simulink model "diastaurosh_31_10_servo_angle"  (R2024b)
settings: Solver=FixedStepDiscrete  StartTime=0.0  StopTime=inf  FixedStep=0.00001  RelTol=1e-3  EnableMultiTasking=on
undefined symbols (not defined in the file): DiscIntNeverNeededParam
libraries: frdmtfcshieldlib x8, slpidlib x4, RHIT_KL25Z_Library x2, Autonomous_Vehicle_Competition x2, frdmkl25zlib x2
settings Model: Creator=maste  LastModifiedBy=kapki
settings SolverCC: AutoInsertRateTranBlk=on  EnableFixedStepZeroCrossing=on
settings DataIOCC: ReturnWorkspaceOutputs=off
settings OptimizationCC: LifeSpan=1  MaxStackSize=64  EfficientTunableParamExpr=on
settings DebuggingCC: ArithmeticOperatorsInVariantConditions=warning
settings HardwareCC: ProdBitPerPointer=32  ProdBitPerSizeT=32  ProdBitPerPtrDiffT=32  ProdLargestAtomicInteger=Long  ProdLargestAtomicFloat=Double  ProdWordSize=32  ProdHWDeviceType=ARM Compatible->ARM Cortex
settings ModelReferenceCC: EnableRefExpFcnMdlSchedulingChecks=on
settings SFSimCC: MATLABDynamicMemAlloc=off  CustomCodeUndefinedFunction=UseInterfaceOnly
settings RTWCC: Description=Embedded Coder  SystemTargetFile=ert.tlc  HardwareBoard=NXP FRDM-KL25Z  TemplateMakefile=ert_default_tmf  Toolchain=GNU Tools for ARM Embedded Processors  GPUComputeCapability=3.5
settings CodeAppCC: IgnoreCustomStorageClasses=off  StateflowObjectComments=on
settings ERTTargetCC: MultiwordLength=2048  SupportContinuousTime=on  InlinedParameterPlacement=Hierarchical  ConvertIfToSwitch=off  SuppressUnreachableDefaultCases=off  DynamicArrayContainerType=coder::array

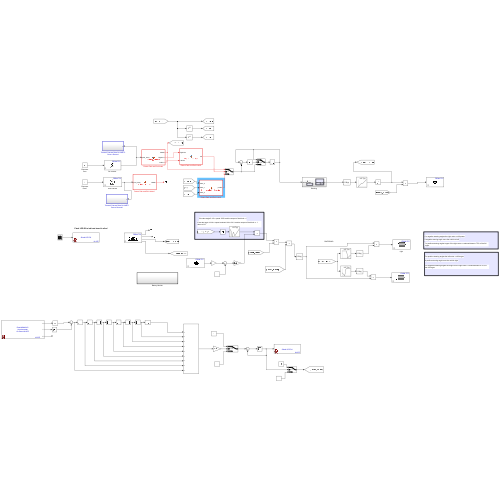
[thumbnail: Simulink's stored preview of the top-level diagram]
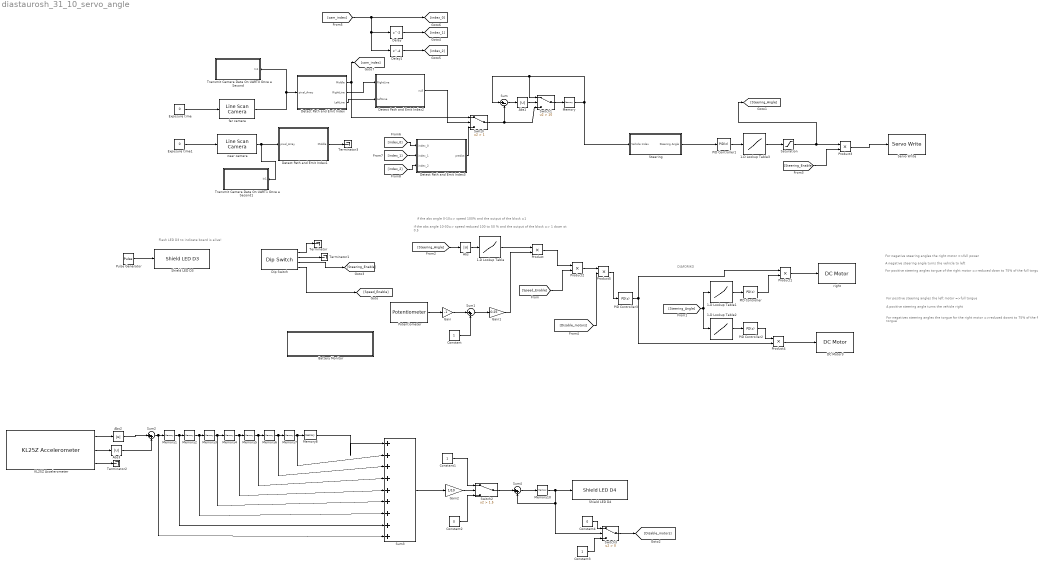
== system diastaurosh_31_10_servo_angle ==
  note: Flash LED D3 to indicate board is alive!
  note: if the abs angle 0-10=> speed 100% and the output of the block =1
  note: if the abs angle 10-30=> speed reduced 100 to 50 % and the output of the block => 1 down ot 0.5
  note: For positive steering angles torgue of the right motor =>reduced down to 75% of the full torgue
  note: For negatives steering angles the torgue for the right motor =>reduced downt to 75% of the full torgue
  note: For positive steering angles the left motor =>full torgue
  note: For negative steering angles the right motor =>full power
  note: A negative steering angle turns the vehicle to left
  note: DIAFORIKO
  note: A positive steering angle turns the vehicle right
  1-D Lookup Table : Lookup_n-D  NumberOfTableDimensions=1  BreakpointsForDimension1="[0  10 20 30 60]"  Table=[ 1.4 0.9 1.2 0.95 1.4]  ExtrapMethod=Clip  UseLastTableValue=on  InternalRulePriority=Speed  RndMeth=Simplest
  1-D Lookup Table1 : Lookup_n-D  NumberOfTableDimensions=1  BreakpointsForDimension1=[-60 0 10 20 60]  Table=[1.1 1.1 1 0.6 0.8]  ExtrapMethod=Clip  UseLastTableValue=on  InternalRulePriority=Speed  RndMeth=Simplest
  1-D Lookup Table2 : Lookup_n-D  NumberOfTableDimensions=1  BreakpointsForDimension1="[-60  -20 -10  0 60]"  Table=[0.8 0.6 1 1.1 1.1]  ExtrapMethod=Clip  UseLastTableValue=on  InternalRulePriority=Speed  RndMeth=Simplest
  1-D Lookup Table3 : Lookup_n-D  NumberOfTableDimensions=1  BreakpointsForDimension1=[-60 -9 9 60]  Table=[-60 0 0 60]  ExtrapMethod=Clip  UseLastTableValue=on  InternalRulePriority=Speed  RndMeth=Simplest
  Abs{,1..3} (4 alike) : Abs  SaturateOnIntegerOverflow=off
  Battery Monitor : Subsystem  TreatAsAtomicUnit=on  SystemSampleTime=0.1
  Constant : Constant
  Constant1 : Constant
  Constant2 : Constant  Value=0
  Constant3 : Constant
  Constant4 : Constant  Value=0
  DC Motor3 : frdmtfcshieldlib/DC Motor  WhichMotor=B
  Delay : Delay  InitialCondition=64
  Delay1 : Delay  DelayLength=4  InitialCondition=64
  Detect Path and Emit Index : MATLAB Function  TreatAsAtomicUnit=on
  Detect Path and Emit Index1 : MATLAB Function  TreatAsAtomicUnit=on
  Detect Path and Emit Index2 : MATLAB Function  TreatAsAtomicUnit=on
  Detect Path and Emit Index3 : MATLAB Function  TreatAsAtomicUnit=on
  Dip Switch : frdmtfcshieldlib/Dip Switch  SampleTime=-1
  Exposure time : Constant  Value=0
  Exposure time1 : Constant  Value=0
  Gain : Gain  Gain=-1
  Gain1 : Gain  Gain=0.25
  Gain2 : Gain  Gain=1/10
  KL25Z Accelerometer : RHIT_KL25Z_Library/Sensor Read Functions/KL25Z Accelerometer
      settings: SourceProductName=RHIT KL25Z Library
  Memory : Memory  InitialCondition=64
  Memory{1..8,10} (9 alike) : Memory
  PID Controller : slpidlib/PID Controller  Controller=PD  Form=Parallel  TimeDomain=Discrete-time  UseExternalTs=off  SampleTime=-1  IntegratorMethod=Forward Euler  FilterMethod=Forward Euler  ControllerParametersSource=internal  P=1  I=1  UseKiTs=off  D=0  UseExternalDerivativeSource=off  N=100  UseFilter=on  TunerSelectOption=Transfer Function Based (PID Tuner App)  InitialConditionSource=internal  InitialConditionForIntegrator=0  InitialConditionForFilter=0  DifferentiatorICPrevScaledInput=0  ExternalReset=none  TrackingMode=off  Kt=1  LimitOutput=off  SatLimitsSource=internal  UpperSaturationLimit=inf  LowerSaturationLimit=-inf  LinearizeAsGain=on  AntiWindupMode=none  Kb=1  LimitIntegrator=off  UpperIntegratorSaturationLimit=inf  LowerIntegratorSaturationLimit=-inf  POutMin=[]  POutMax=[]  IOutMin=[]  IOutMax=[]  DOutMin=[]  DOutMax=[]  NOutMin=[]  NOutMax=[]  SumOutMin=[]  SumOutMax=[]  SaturationOutMin=[]  SaturationOutMax=[]  PParamMin=[]  PParamMax=[]  IParamMin=[]  IParamMax=[]  DParamMin=[]  DParamMax=[]  NParamMin=[]  NParamMax=[]  KbParamMin=[]  KbParamMax=[]  KtParamMin=[]  KtParamMax=[]  KbOutMin=[]  KbOutMax=[]  KtOutMin=[]  KtOutMax=[]  IntegratorOutMin=[]  IntegratorOutMax=[]  FilterOutMin=[]  FilterOutMax=[]  SumI1OutMin=[]  SumI1OutMax=[]  SumI2OutMin=[]  SumI2OutMax=[]  SumI3OutMin=[]  SumI3OutMax=[]  SumI4OutMin=[]  SumI4OutMax=[]  SumDOutMin=[]  SumDOutMax=[]  DifferentiatorOutMin=[]  DifferentiatorOutMax=[]  FilterDiffOutCoefMin=[]  FilterDiffOutCoefMax=[]  ReciprocalOutMin=[]  ReciprocalOutMax=[]  SumDenOutMin=[]  SumDenOutMax=[]  SumNumOutMin=[]  SumNumOutMax=[]  DivideOutMin=[]  DivideOutMax=[]  UdiffTsProdOutMin=[]  UdiffTsProdOutMax=[]  NTsProdOutMin=[]  NTsProdOutMax=[]  UintegralTsProdOutMin=[]  UintegralTsProdOutMax=[]  UngainTsProdOutMin=[]  UngainTsProdOutMax=[]  ClampingZeroOutDataTypeStr=Inherit: Inherit via back propagation  ClampingZeroOutMin=[]  ClampingZeroOutMax=[]  FilterDenConstantOutDataTypeStr=Inherit: Inherit via back propagation  FilterDenConstantOutMin=[]  FilterDenConstantOutMax=[]  PCopyOutDataTypeStr=Inherit: Inherit via back propagation  PCopyOutMin=[]  PCopyOutMax=[]  NCopyOutDataTypeStr=Inherit: Inherit via back propagation  NCopyOutMin=[]  NCopyOutMax=[]  IntegratorContinuousStateAttributes=''  IntegratorStateMustResolveToSignalObject=off  IntegratorRTWStateStorageClass=Auto  FilterContinuousStateAttributes=''  FilterStateMustResolveToSignalObject=off  FilterRTWStateStorageClass=Auto  ParallelPVariant=InternalParameters  IdealPVariant=Disabled  IVariant=Disabled  DVariant=InternalParameters  IntegratorVariant=Disabled  SatVariant=Disabled  AWVariant=Disabled  PCopyVariant=Disabled  TRVariant=Disabled  FdbkBlocksVariant=Forward  IdealPFdbkVariant=Disabled  SatFdbkVariant=Disabled  DerivativeFilterVariant=ForwardEulerFilter  NVariant=InternalParameters  NCopyVariant=Disabled  FilterICVariant=InternalICsFilter  IntegratorICVariant=Disabled  ExternalResetVariant=Disabled  TRSumVariant=Passthrough  SumFdbkVariant=Disabled  SumVariant=Sum_PD  TsampFilterVariant=InternalTs  TsampNgainVariant=Passthrough  TsampIntegralVariant=Disabled_SignalSpec  ExternalSaturationOutDataTypeStr=Inherit: Same as second input  DerivativeSourceVariant=ErrorSignal  PreIntVariant=InternalPreInt
  PID Controller1 : slpidlib/PID Controller  Controller=PID  Form=Parallel  TimeDomain=Discrete-time  UseExternalTs=off  SampleTime=-1  IntegratorMethod=Forward Euler  FilterMethod=Forward Euler  ControllerParametersSource=internal  P=1  I=1.1  UseKiTs=off  D=0  UseExternalDerivativeSource=off  N=70  UseFilter=on  TunerSelectOption=Transfer Function Based (PID Tuner App)  InitialConditionSource=internal  InitialConditionForIntegrator=0  InitialConditionForFilter=0  DifferentiatorICPrevScaledInput=0  ExternalReset=none  TrackingMode=off  Kt=1  LimitOutput=off  SatLimitsSource=internal  UpperSaturationLimit=inf  LowerSaturationLimit=-inf  LinearizeAsGain=on  AntiWindupMode=none  Kb=1  LimitIntegrator=off  UpperIntegratorSaturationLimit=inf  LowerIntegratorSaturationLimit=-inf  POutMin=[]  POutMax=[]  IOutMin=[]  IOutMax=[]  DOutMin=[]  DOutMax=[]  NOutMin=[]  NOutMax=[]  SumOutMin=[]  SumOutMax=[]  SaturationOutMin=[]  SaturationOutMax=[]  PParamMin=[]  PParamMax=[]  IParamMin=[]  IParamMax=[]  DParamMin=[]  DParamMax=[]  NParamMin=[]  NParamMax=[]  KbParamMin=[]  KbParamMax=[]  KtParamMin=[]  KtParamMax=[]  KbOutMin=[]  KbOutMax=[]  KtOutMin=[]  KtOutMax=[]  IntegratorOutMin=[]  IntegratorOutMax=[]  FilterOutMin=[]  FilterOutMax=[]  SumI1OutMin=[]  SumI1OutMax=[]  SumI2OutMin=[]  SumI2OutMax=[]  SumI3OutMin=[]  SumI3OutMax=[]  SumI4OutMin=[]  SumI4OutMax=[]  SumDOutMin=[]  SumDOutMax=[]  DifferentiatorOutMin=[]  DifferentiatorOutMax=[]  FilterDiffOutCoefMin=[]  FilterDiffOutCoefMax=[]  ReciprocalOutMin=[]  ReciprocalOutMax=[]  SumDenOutMin=[]  SumDenOutMax=[]  SumNumOutMin=[]  SumNumOutMax=[]  DivideOutMin=[]  DivideOutMax=[]  UdiffTsProdOutMin=[]  UdiffTsProdOutMax=[]  NTsProdOutMin=[]  NTsProdOutMax=[]  UintegralTsProdOutMin=[]  UintegralTsProdOutMax=[]  UngainTsProdOutMin=[]  UngainTsProdOutMax=[]  ClampingZeroOutDataTypeStr=Inherit: Inherit via back propagation  ClampingZeroOutMin=[]  ClampingZeroOutMax=[]  FilterDenConstantOutDataTypeStr=Inherit: Inherit via back propagation  FilterDenConstantOutMin=[]  FilterDenConstantOutMax=[]  PCopyOutDataTypeStr=Inherit: Inherit via back propagation  PCopyOutMin=[]  PCopyOutMax=[]  NCopyOutDataTypeStr=Inherit: Inherit via back propagation  NCopyOutMin=[]  NCopyOutMax=[]  IntegratorContinuousStateAttributes=''  IntegratorStateMustResolveToSignalObject=off  IntegratorRTWStateStorageClass=Auto  FilterContinuousStateAttributes=''  FilterStateMustResolveToSignalObject=off  FilterRTWStateStorageClass=Auto  ParallelPVariant=InternalParameters  IdealPVariant=Disabled  IVariant=InternalParameters  DVariant=InternalParameters  IntegratorVariant=Discrete  SatVariant=Disabled  AWVariant=Passthrough  PCopyVariant=Disabled  TRVariant=Disabled  FdbkBlocksVariant=Forward  IdealPFdbkVariant=Disabled  SatFdbkVariant=Disabled  DerivativeFilterVariant=ForwardEulerFilter  NVariant=InternalParameters  NCopyVariant=Disabled  FilterICVariant=InternalICsFilter  IntegratorICVariant=InternalICs  ExternalResetVariant=Disabled  TRSumVariant=Passthrough  SumFdbkVariant=Disabled  SumVariant=Sum_PID  TsampFilterVariant=InternalTs  TsampNgainVariant=Passthrough  TsampIntegralVariant=Disabled_SignalSpec  ExternalSaturationOutDataTypeStr=Inherit: Same as second input  DerivativeSourceVariant=ErrorSignal  PreIntVariant=InternalPreInt
  PID Controller2 : slpidlib/PID Controller  Controller=PD  Form=Parallel  TimeDomain=Discrete-time  UseExternalTs=off  SampleTime=-1  IntegratorMethod=Forward Euler  FilterMethod=Forward Euler  ControllerParametersSource=internal  P=1  I=1  UseKiTs=off  D=0  UseExternalDerivativeSource=off  N=100  UseFilter=on  TunerSelectOption=Transfer Function Based (PID Tuner App)  InitialConditionSource=internal  InitialConditionForIntegrator=0  InitialConditionForFilter=0  DifferentiatorICPrevScaledInput=0  ExternalReset=none  TrackingMode=off  Kt=1  LimitOutput=off  SatLimitsSource=internal  UpperSaturationLimit=inf  LowerSaturationLimit=-inf  LinearizeAsGain=on  AntiWindupMode=none  Kb=1  LimitIntegrator=off  UpperIntegratorSaturationLimit=inf  LowerIntegratorSaturationLimit=-inf  POutMin=[]  POutMax=[]  IOutMin=[]  IOutMax=[]  DOutMin=[]  DOutMax=[]  NOutMin=[]  NOutMax=[]  SumOutMin=[]  SumOutMax=[]  SaturationOutMin=[]  SaturationOutMax=[]  PParamMin=[]  PParamMax=[]  IParamMin=[]  IParamMax=[]  DParamMin=[]  DParamMax=[]  NParamMin=[]  NParamMax=[]  KbParamMin=[]  KbParamMax=[]  KtParamMin=[]  KtParamMax=[]  KbOutMin=[]  KbOutMax=[]  KtOutMin=[]  KtOutMax=[]  IntegratorOutMin=[]  IntegratorOutMax=[]  FilterOutMin=[]  FilterOutMax=[]  SumI1OutMin=[]  SumI1OutMax=[]  SumI2OutMin=[]  SumI2OutMax=[]  SumI3OutMin=[]  SumI3OutMax=[]  SumI4OutMin=[]  SumI4OutMax=[]  SumDOutMin=[]  SumDOutMax=[]  DifferentiatorOutMin=[]  DifferentiatorOutMax=[]  FilterDiffOutCoefMin=[]  FilterDiffOutCoefMax=[]  ReciprocalOutMin=[]  ReciprocalOutMax=[]  SumDenOutMin=[]  SumDenOutMax=[]  SumNumOutMin=[]  SumNumOutMax=[]  DivideOutMin=[]  DivideOutMax=[]  UdiffTsProdOutMin=[]  UdiffTsProdOutMax=[]  NTsProdOutMin=[]  NTsProdOutMax=[]  UintegralTsProdOutMin=[]  UintegralTsProdOutMax=[]  UngainTsProdOutMin=[]  UngainTsProdOutMax=[]  ClampingZeroOutDataTypeStr=Inherit: Inherit via back propagation  ClampingZeroOutMin=[]  ClampingZeroOutMax=[]  FilterDenConstantOutDataTypeStr=Inherit: Inherit via back propagation  FilterDenConstantOutMin=[]  FilterDenConstantOutMax=[]  PCopyOutDataTypeStr=Inherit: Inherit via back propagation  PCopyOutMin=[]  PCopyOutMax=[]  NCopyOutDataTypeStr=Inherit: Inherit via back propagation  NCopyOutMin=[]  NCopyOutMax=[]  IntegratorContinuousStateAttributes=''  IntegratorStateMustResolveToSignalObject=off  IntegratorRTWStateStorageClass=Auto  FilterContinuousStateAttributes=''  FilterStateMustResolveToSignalObject=off  FilterRTWStateStorageClass=Auto  ParallelPVariant=InternalParameters  IdealPVariant=Disabled  IVariant=Disabled  DVariant=InternalParameters  IntegratorVariant=Disabled  SatVariant=Disabled  AWVariant=Disabled  PCopyVariant=Disabled  TRVariant=Disabled  FdbkBlocksVariant=Forward  IdealPFdbkVariant=Disabled  SatFdbkVariant=Disabled  DerivativeFilterVariant=ForwardEulerFilter  NVariant=InternalParameters  NCopyVariant=Disabled  FilterICVariant=InternalICsFilter  IntegratorICVariant=Disabled  ExternalResetVariant=Disabled  TRSumVariant=Passthrough  SumFdbkVariant=Disabled  SumVariant=Sum_PD  TsampFilterVariant=InternalTs  TsampNgainVariant=Passthrough  TsampIntegralVariant=Disabled_SignalSpec  ExternalSaturationOutDataTypeStr=Inherit: Same as second input  DerivativeSourceVariant=ErrorSignal  PreIntVariant=InternalPreInt
  PID Controller3 : slpidlib/PID Controller  Controller=PD  Form=Parallel  TimeDomain=Discrete-time  UseExternalTs=off  SampleTime=-1  IntegratorMethod=Forward Euler  FilterMethod=Forward Euler  ControllerParametersSource=internal  P=1  I=1  UseKiTs=off  D=0  UseExternalDerivativeSource=off  N=100  UseFilter=on  TunerSelectOption=Transfer Function Based (PID Tuner App)  InitialConditionSource=internal  InitialConditionForIntegrator=0  InitialConditionForFilter=0  DifferentiatorICPrevScaledInput=0  ExternalReset=none  TrackingMode=off  Kt=1  LimitOutput=off  SatLimitsSource=internal  UpperSaturationLimit=inf  LowerSaturationLimit=-inf  LinearizeAsGain=on  AntiWindupMode=none  Kb=1  LimitIntegrator=off  UpperIntegratorSaturationLimit=inf  LowerIntegratorSaturationLimit=-inf  POutMin=[]  POutMax=[]  IOutMin=[]  IOutMax=[]  DOutMin=[]  DOutMax=[]  NOutMin=[]  NOutMax=[]  SumOutMin=[]  SumOutMax=[]  SaturationOutMin=[]  SaturationOutMax=[]  PParamMin=[]  PParamMax=[]  IParamMin=[]  IParamMax=[]  DParamMin=[]  DParamMax=[]  NParamMin=[]  NParamMax=[]  KbParamMin=[]  KbParamMax=[]  KtParamMin=[]  KtParamMax=[]  KbOutMin=[]  KbOutMax=[]  KtOutMin=[]  KtOutMax=[]  IntegratorOutMin=[]  IntegratorOutMax=[]  FilterOutMin=[]  FilterOutMax=[]  SumI1OutMin=[]  SumI1OutMax=[]  SumI2OutMin=[]  SumI2OutMax=[]  SumI3OutMin=[]  SumI3OutMax=[]  SumI4OutMin=[]  SumI4OutMax=[]  SumDOutMin=[]  SumDOutMax=[]  DifferentiatorOutMin=[]  DifferentiatorOutMax=[]  FilterDiffOutCoefMin=[]  FilterDiffOutCoefMax=[]  ReciprocalOutMin=[]  ReciprocalOutMax=[]  SumDenOutMin=[]  SumDenOutMax=[]  SumNumOutMin=[]  SumNumOutMax=[]  DivideOutMin=[]  DivideOutMax=[]  UdiffTsProdOutMin=[]  UdiffTsProdOutMax=[]  NTsProdOutMin=[]  NTsProdOutMax=[]  UintegralTsProdOutMin=[]  UintegralTsProdOutMax=[]  UngainTsProdOutMin=[]  UngainTsProdOutMax=[]  ClampingZeroOutDataTypeStr=Inherit: Inherit via back propagation  ClampingZeroOutMin=[]  ClampingZeroOutMax=[]  FilterDenConstantOutDataTypeStr=Inherit: Inherit via back propagation  FilterDenConstantOutMin=[]  FilterDenConstantOutMax=[]  PCopyOutDataTypeStr=Inherit: Inherit via back propagation  PCopyOutMin=[]  PCopyOutMax=[]  NCopyOutDataTypeStr=Inherit: Inherit via back propagation  NCopyOutMin=[]  NCopyOutMax=[]  IntegratorContinuousStateAttributes=''  IntegratorStateMustResolveToSignalObject=off  IntegratorRTWStateStorageClass=Auto  FilterContinuousStateAttributes=''  FilterStateMustResolveToSignalObject=off  FilterRTWStateStorageClass=Auto  ParallelPVariant=InternalParameters  IdealPVariant=Disabled  IVariant=Disabled  DVariant=InternalParameters  IntegratorVariant=Disabled  SatVariant=Disabled  AWVariant=Disabled  PCopyVariant=Disabled  TRVariant=Disabled  FdbkBlocksVariant=Forward  IdealPFdbkVariant=Disabled  SatFdbkVariant=Disabled  DerivativeFilterVariant=ForwardEulerFilter  NVariant=InternalParameters  NCopyVariant=Disabled  FilterICVariant=InternalICsFilter  IntegratorICVariant=Disabled  ExternalResetVariant=Disabled  TRSumVariant=Passthrough  SumFdbkVariant=Disabled  SumVariant=Sum_PD  TsampFilterVariant=InternalTs  TsampNgainVariant=Passthrough  TsampIntegralVariant=Disabled_SignalSpec  ExternalSaturationOutDataTypeStr=Inherit: Same as second input  DerivativeSourceVariant=ErrorSignal  PreIntVariant=InternalPreInt
  Potentiometer : frdmtfcshieldlib/Potentiometer  WhichPot=A  SampleTime=-1
  Product{,1..5} (6 alike) : Product
  Pulse Generator : DiscretePulseGenerator  PulseType=Time based  Period=10  PulseWidth=5
  Saturation : Saturate  UpperLimit=45  LowerLimit=-45
  Servo Write : frdmtfcshieldlib/Servo Write  WhichServo=0  minAngle=-45  maxAngle=45
  Shield LED D3 : Autonomous_Vehicle_Competition/Shield LED D3
      settings: SourceProductName=Autonomous Vehicle Competition
  Shield LED D4 : Autonomous_Vehicle_Competition/Shield LED D4
      settings: SourceProductName=Autonomous Vehicle Competition
  Steering : Subsystem
  Sum : Sum  Inputs=|+-
  Sum1 : Sum  Inputs=|++
  Sum2 : Sum  Inputs=|++
  Sum3 : Sum  Inputs=|+++++++++
  Sum4 : Sum  Inputs=|++
  Switch : Switch  Criteria=u2 > Threshold  Threshold=1  SaturateOnIntegerOverflow=off  InputSameDT=off
  Switch1 : Switch  Criteria=u2 > Threshold  Threshold=10  SaturateOnIntegerOverflow=off  InputSameDT=off
  Switch2 : Switch  Criteria=u2 > Threshold  Threshold=1.5  SaturateOnIntegerOverflow=off  InputSameDT=off
  Switch3 : Switch  Criteria=u2 > Threshold  SaturateOnIntegerOverflow=off  InputSameDT=off
  Terminator{,1..3} (4 alike) : Terminator
  Transmit Camera Data On UART0 Once a Second : Subsystem  TreatAsAtomicUnit=on  SystemSampleTime=.26
  Transmit Camera Data On UART1 Once a Second1 : Subsystem  TreatAsAtomicUnit=on  SystemSampleTime=.26
  "far camera " : frdmtfcshieldlib/Line Scan Camera  CameraHeader=0  SampleTime=0.00001
  near camera : frdmtfcshieldlib/Line Scan Camera  CameraHeader=1  SampleTime=0.00001
  right : frdmtfcshieldlib/DC Motor  WhichMotor=A
  wires:
  Exposure time/1 -> "far camera "/1
  "far camera "/1 -> Transmit Camera Data On UART0 Once a Second/1(In1), Detect Path and Emit Index/1(pixel_Array)
  1-D Lookup Table/1 -> Product/1
  Gain1/1 -> Product/2
  [Steering_Angle] -> Abs/1
  Abs/1 -> 1-D Lookup Table/1
  Pulse Generator/1 -> Shield LED D3/1
  [Steering_Angle] -> 1-D Lookup Table2/1, 1-D Lookup Table1/1
  1-D Lookup Table1/1 -> PID Controller/1
  PID Controller/1 -> Product1/2
  1-D Lookup Table2/1 -> PID Controller2/1
  PID Controller2/1 -> Product4/1
  PID Controller3/1 -> Product4/2, Product1/1
  1-D Lookup Table3/1 -> Saturation/1
  Product1/1 -> right/1
  Product4/1 -> DC Motor3/1
  Dip Switch/1 -> Terminator/1
  Dip Switch/2 -> Terminator1/1
  Product/1 -> Product2/1
  [Speed_Enable] -> Product2/2
  Product3/1 -> Servo Write/1
  [Steering_Enable] -> Product3/2
  Dip Switch/4 -> [Speed_Enable]
  Dip Switch/3 -> [Steering_Enable]
  Steering/1(Steering Angle) -> PID Controller1/1
  PID Controller1/1 -> 1-D Lookup Table3/1
  Saturation/1 -> Product3/1, [Steering_Angle]
  Exposure time1/1 -> near camera/1
  near camera/1 -> Transmit Camera Data On UART1 Once a Second1/1(In1), Detect Path and Emit Index1/1(pixel_Array)
  Detect Path and Emit Index2/1(null) -> Switch/2
  Detect Path and Emit Index/1(Middle) -> [cam_index], Switch/1
  Detect Path and Emit Index/2(RightLine) -> Detect Path and Emit Index2/1(RightLine)
  Detect Path and Emit Index/3(LeftLine) -> Detect Path and Emit Index2/2(LeftLine)
  Memory/1 -> Steering/1(Vehicle Index), Switch1/1, Sum/1
  Abs1/1 -> Switch1/2
  Switch1/1 -> Memory/1
  Switch/1 -> Sum/2, Switch1/3
  Sum/1 -> Abs1/1
  Potentiometer/1 -> Gain/1
  Gain/1 -> Sum1/1
  Constant/1 -> Sum1/2
  Sum1/1 -> Gain1/1
  KL25Z Accelerometer/3 -> Terminator2/1
  KL25Z Accelerometer/1 -> Abs2/1
  KL25Z Accelerometer/2 -> Abs3/1
  Abs3/1 -> Sum2/2
  Abs2/1 -> Sum2/1
  Memory1/1 -> Sum3/8, Memory2/1
  Sum2/1 -> Sum3/9, Memory1/1
  Memory2/1 -> Sum3/7, Memory3/1
  Memory3/1 -> Sum3/6, Memory4/1
  Memory4/1 -> Sum3/5, Memory5/1
  Memory5/1 -> Sum3/4, Memory6/1
  Memory6/1 -> Sum3/3, Memory7/1
  Memory7/1 -> Sum3/2, Memory8/1
  Memory8/1 -> Sum3/1
  Sum3/1 -> Gain2/1
  Constant1/1 -> Switch2/1
  Constant2/1 -> Switch2/3
  Gain2/1 -> Switch2/2
  Switch2/1 -> Sum4/1
  Memory10/1 -> Shield LED D4/1, Switch3/2, Sum4/2
  Sum4/1 -> Memory10/1
  Constant4/1 -> Switch3/1
  Constant3/1 -> Switch3/3
  Switch3/1 -> [Disable_motors]
  Product2/1 -> Product5/1
  Product5/1 -> PID Controller3/1
  [Disable_motors] -> Product5/2
  Delay/1 -> [index_1]
  Delay1/1 -> [index_2]
  [cam_index] -> [index_0], Delay/1, Delay1/1
  [index_0] -> Detect Path and Emit Index3/1(index_0)
  [index_1] -> Detect Path and Emit Index3/2(index_1)
  [index_2] -> Detect Path and Emit Index3/3(index_2)
  Detect Path and Emit Index3/1(predict) -> Switch/3
  Detect Path and Emit Index1/1(Middle) -> Terminator3/1

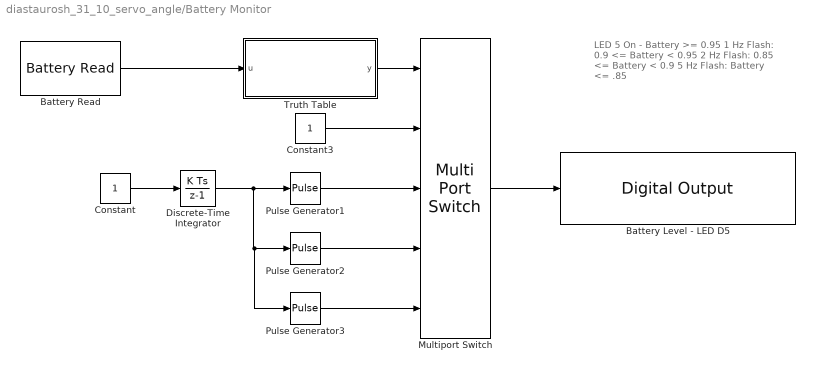
== system diastaurosh_31_10_servo_angle/Battery Monitor ==
  note: LED 5
      | On - Battery >= 0.95
      | 1 Hz Flash: 0.9 <= Battery < 0.95
      | 2 Hz Flash: 0.85 <= Battery < 0.9
      | 5 Hz Flash: Battery <= .85
  Battery Level - LED D5 : RHIT_KL25Z_Library/Basic Blocks/Digital Output  WhichPin=PTB10
      settings: SourceProductName=RHIT KL25Z Library
  Battery Read : frdmtfcshieldlib/Battery Read  SampleTime=-1
  Constant : Constant
  Constant3 : Constant  OutDataTypeStr=single
  Discrete-Time Integrator : DiscreteIntegrator  SampleTime=-1  ICPrevOutput=DiscIntNeverNeededParam  ICPrevScaledInput=DiscIntNeverNeededParam
  Multiport Switch : MultiPortSwitch  Inputs=4  SaturateOnIntegerOverflow=off  InputSameDT=off
  Pulse Generator1 : DiscretePulseGenerator  PulseType=Time based  TimeSource=Use external signal  Period=1  PulseWidth=50
  Pulse Generator2 : DiscretePulseGenerator  PulseType=Time based  TimeSource=Use external signal  Period=.5  PulseWidth=60
  Pulse Generator3 : DiscretePulseGenerator  PulseType=Time based  TimeSource=Use external signal  Period=.2  PulseWidth=50
  Truth Table : Truth Table  TreatAsAtomicUnit=on
  wires:
  Pulse Generator2/1 -> Multiport Switch/4
  Truth Table/1(y) -> Multiport Switch/1
  Pulse Generator1/1 -> Multiport Switch/3
  Constant3/1 -> Multiport Switch/2
  Battery Read/1 -> Truth Table/1(u)
  Pulse Generator3/1 -> Multiport Switch/5
  Multiport Switch/1 -> Battery Level - LED D5/1
  Discrete-Time Integrator/1 -> Pulse Generator3/1, Pulse Generator2/1, Pulse Generator1/1
  Constant/1 -> Discrete-Time Integrator/1

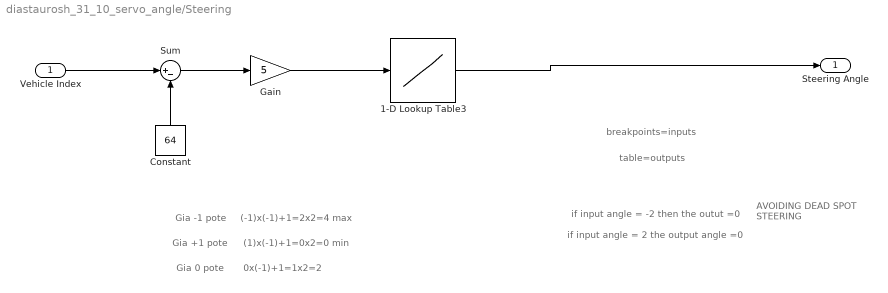
== system diastaurosh_31_10_servo_angle/Steering ==
  note: AVOIDING
      | DEAD SPOT STEERING
  note: if input angle = 2 the output angle =0
  note: if input angle = -2 then the outut =0
  note: table=outputs
  note: breakpoints=inputs
  note: 0x(-1)+1=1x2=2
  note: Gia 0 pote
  note: Gia +1 pote
  note: Gia -1 pote
  note: (1)x(-1)+1=0x2=0 min
  note: (-1)x(-1)+1=2x2=4 max
  Vehicle Index : Inport
  1-D Lookup Table3 : Lookup_n-D  NumberOfTableDimensions=1  BreakpointsForDimension1=[-60 -9 9 60]  Table=[-60 0 0 60]  ExtrapMethod=Clip  UseLastTableValue=on  InternalRulePriority=Speed  RndMeth=Simplest
  Constant : Constant  Value=64
  Gain : Gain  Gain=5
  Sum : Sum  Inputs=|+-
  Steering Angle : Outport
  wires:
  Constant/1 -> Sum/2
  Vehicle Index/1 -> Sum/1
  Gain/1 -> 1-D Lookup Table3/1
  Sum/1 -> Gain/1
  1-D Lookup Table3/1 -> Steering Angle/1

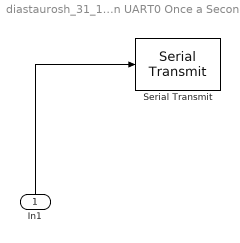
== system diastaurosh_31_10_servo_angle/Transmit Camera Data On UART0 Once a Second ==
  In1 : Inport
  Serial Transmit : frdmkl25zlib/Serial Transmit  uart=UART0  sendmode=printf
  wires:
  In1/1 -> Serial Transmit/1

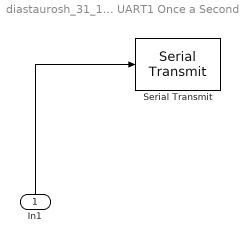
== system diastaurosh_31_10_servo_angle/Transmit Camera Data On UART1 Once a Second1 ==
  In1 : Inport
  Serial Transmit : frdmkl25zlib/Serial Transmit  uart=UART1  sendmode=printf
  wires:
  In1/1 -> Serial Transmit/1

== matlab function diastaurosh_31_10_servo_angle/Battery Monitor/Truth Table ==
  data: u input; y output
function y = fcn(u)

aVarTruthTableCondition_1 = false;
aVarTruthTableCondition_2 = false;
aVarTruthTableCondition_3 = false;


% Fully Charged

aVarTruthTableCondition_1 = logical(u >= 0.95);

% Low

aVarTruthTableCondition_2 = logical(u>=0.9);

% Lower

aVarTruthTableCondition_3 = logical(u>=.85);

if (aVarTruthTableCondition_1 && aVarTruthTableCondition_2 && aVarTruthTableCondition_3)
    aFcnTruthTableAction_1();
elseif (~aVarTruthTableCondition_1 && aVarTruthTableCondition_2 && aVarTruthTableCondition_3)
    aFcnTruthTableAction_2();
elseif (~aVarTruthTableCondition_1 && ~aVarTruthTableCondition_2 && aVarTruthTableCondition_3)
    aFcnTruthTableAction_3();
elseif (~aVarTruthTableCondition_1 && ~aVarTruthTableCondition_2 && ~aVarTruthTableCondition_3)
    aFcnTruthTableAction_4();
else % Default
    aFcnTruthTableAction_4();
end

function aFcnTruthTableAction_1()

% Fully Charged

y=1;

function aFcnTruthTableAction_2()

% Low 1

y=2;

function aFcnTruthTableAction_3()

% lOW 2

y=3;

function aFcnTruthTableAction_4()

% Dead

y=4;

== matlab function diastaurosh_31_10_servo_angle/Detect Path and Emit Index ==
  data: Middle output single; pixel_Array input; RightLine output; LeftLine output
  function [Middle,RightLine,LeftLine] = Steering_Function(pixel_Array)
  
    % Initialize variables
    LeftLine = single(1);
    RightLine = single(127);
  
   thresh = 0.75 * mean(pixel_Array(40:80));
    
    % Find LeftLine
    for i = 63:-1:1
        if pixel_Array(i) < thresh
            LeftLine = single(i);
            break;
        end
    end

    % Find RightLine
    for i = 64:127
        if pixel_Array(i) < thresh
            RightLine = single(i);
            break;
        end
    end
  
  Middle = (RightLine + LeftLine) / 2;
  if RightLine > 120
      Middle = LeftLine + 64;
  end
  if LeftLine < 6
      Middle = RightLine - 64;
  

  end
      
  end

== matlab function diastaurosh_31_10_servo_angle/Detect Path and Emit Index1 ==
  data: Middle output single; pixel_Array input
function Middle = Steering_Function(pixel_Array)
    % Initialize variables
    LeftLine = single(1);
    RightLine = single(127);
    Middle=single(64);
  
    thresh = 0.75 * mean(pixel_Array(40:80));
    
    % Find LeftLine
    for i = 63:-1:1
        if pixel_Array(i) < thresh
            LeftLine = single(i);
            break;
        end
    end

    % Find RightLine
    for i = 64:127
        if pixel_Array(i) < thresh
            RightLine = single(i);
            break;
        end
    end
    
    % Calculate Middle based on conditions
    if RightLine > 120
        Middle = LeftLine + 67;
    elseif LeftLine < 6
        Middle = RightLine - 67;
    elseif RightLine < 128 && LeftLine > 1
        Middle = (RightLine + LeftLine) / 2;
  
    end
end

== matlab function diastaurosh_31_10_servo_angle/Detect Path and Emit Index2 ==
  data: null output single; RightLine input; LeftLine input
function null = Steering_Function( RightLine, LeftLine)
                    % Array to store the LineScan image

                    if RightLine>120 && LeftLine<6
                        null=single(2);
                        
                    else
                        null=single(0);
                    end 
                    end

== matlab function diastaurosh_31_10_servo_angle/Detect Path and Emit Index3 ==
  data: predict output single; index_0 input; index_1 input; index_2 input
function predict = index_prediction_Function(index_0,index_1,index_2)

delta1 = index_0 - index_1;
delta2 = index_1 - index_2;
avg_delta = (delta1 - delta2)/2;

predict = index_0 + avg_delta;
